simulink model "DDCU_wxt_v02_forA_LabviewV03"  (R2014a)
settings: Solver=FixedStepDiscrete  StartTime=0.0  StopTime=50  FixedStep=0.0005  RelTol=1e-3
InitFcn:
  | Veh_Par_wxt
values from neighbouring files (symbols this model uses):
  ag_thr = 0.4*g    (= 3.924)    [Veh_Par_wxt.m]
  B = 2.25    [Veh_Par_wxt.m]
  bra_pre_em = 12    [Veh_Par_wxt.m]
  bra_pre_gz2 = 12/3    (= 4)    [Veh_Par_wxt.m]
  bra_pre_gz34 = 12/3    (= 4)    [Veh_Par_wxt.m]
  bra_pre_yd = 12/2    (= 6)    [Veh_Par_wxt.m]
  brakepre_dem_data = [0 1 2 3 4 5 6 7 8 9 10 11 12]    [Veh_Par_wxt.m]
  brakeTrq_dem_data = [0 218.198 436.396 654.594 872.792 1090.99 1309.188 1527.386 1745.584 1963.782 2181.98 2400.178 2618.376]    [Veh_Par_wxt.m]
  bratrq_max = 4*2618.376    (= 10473.504)    [Veh_Par_wxt.m]
  eff_tran = 0.75    [Veh_Par_wxt.m]
  G = Mass*g    (= 36297)    [Veh_Par_wxt.m]
  kd1 = 1    [Veh_Par_wxt.m]
  kd2 = 1    [Veh_Par_wxt.m]
  kd3 = 1    [Veh_Par_wxt.m]
  ki1 = 1    [Veh_Par_wxt.m]
  ki2 = 1    [Veh_Par_wxt.m]
  ki3 = 1    [Veh_Par_wxt.m]
  kp1 = 1    [Veh_Par_wxt.m]
  kp2 = 1    [Veh_Par_wxt.m]
  kp3 = 1    [Veh_Par_wxt.m]
  L = 3.12    [Veh_Par_wxt.m]
  premax = 12    [Veh_Par_wxt.m]
  Radius = 0.20    (= 0.2)    [Veh_Par_wxt.m]
  s_opt_yi_add = 0.05    [Veh_Par_wxt.m]
  s_opt_zhuan_add = 0.05    [Veh_Par_wxt.m]
  spd_map_mot = [0 100 200 300 360 400 500 600 700 800 900]*tras_ratio    [Veh_Par_wxt.m]
  spdmax = 900*tras_ratio    (= 5580)    [Veh_Par_wxt.m]
  speed_thr_park = 5/3.6/Radius*30/pi    (= 66.3145596216)    [Veh_Par_wxt.m]
  tras_ratio = 6.2    [Veh_Par_wxt.m]
  trq_map_mot = [1200 1200 1200 1200 1200 1080 864 720 617 540 480]/tras_ratio    [Veh_Par_wxt.m]
  trqmax = 80    [Veh_Par_wxt.m]
  trqmax_yd = 200    [Veh_Par_wxt.m]
  v_thr1_b = 5    [Veh_Par_wxt.m]
  v_thr2_b = 20    [Veh_Par_wxt.m]
  v_thr_park = 5    [Veh_Par_wxt.m]
undefined symbols (not defined in the file or in its folder): DiscIntNeverNeededParam
libraries: simulink x231, ec5744lib x19
(part 9 of 16)

== system DDCU_wxt_v02_forA_LabviewV03/OutputSignalProcess/VCU_MCU2_replace/M4Drive ==
  M4Drive : Inport
  Constant{1..4,6..8} (7 alike) : Constant  Value=0  OutDataTypeStr=uint8
  M4DriveRon : Rounding  Operator=round
  M4Drive_1sat : Saturate  UpperLimit=12  LowerLimit=0
  M4Drive_Convert : DataTypeConversion  OutDataTypeStr=uint8
  M4Drive_Convert1 : DataTypeConversion  OutDataTypeStr=uint32
  M4Drive_D : Product  Inputs=*/
  M4Drive_F : Constant  OutDataTypeStr=single
  M4Drive_L : simulink/Logic and Bit Operations/Bitwise Operator  logicop=AND  UseBitMask=on  BitMask=12  BitMaskRealWorld=Stored Integer
  M4Drive_O : Constant  Value=0  OutDataTypeStr=single
  M4Drive_S : ArithShift  BitShiftNumber=-2
  M4Drive_sat : Saturate  UpperLimit=3  LowerLimit=0
  M4Drive_st : Sum  Inputs=+-
  output1 : Outport
  output2 : Outport  Port=2
  output3 : Outport  Port=3
  output4 : Outport  Port=4
  output5 : Outport  Port=5
  output6 : Outport  Port=6
  output7 : Outport  Port=7
  output8 : Outport  Port=8
  wires:
  M4Drive/1 -> M4Drive_sat/1
  M4Drive_sat/1 -> M4Drive_st/1
  M4Drive_O/1 -> M4Drive_st/2
  M4Drive_st/1 -> M4Drive_D/1
  M4Drive_F/1 -> M4Drive_D/2
  M4Drive_D/1 -> M4DriveRon/1
  M4DriveRon/1 -> M4Drive_S/1
  M4Drive_S/1 -> M4Drive_1sat/1
  M4Drive_1sat/1 -> M4Drive_Convert1/1
  M4Drive_Convert1/1 -> M4Drive_L/1
  M4Drive_L/1 -> M4Drive_Convert/1
  M4Drive_Convert/1 -> output5/1
  Constant1/1 -> output1/1
  Constant2/1 -> output2/1
  Constant3/1 -> output3/1
  Constant4/1 -> output4/1
  Constant6/1 -> output6/1
  Constant7/1 -> output7/1
  Constant8/1 -> output8/1

== system DDCU_wxt_v02_forA_LabviewV03/OutputSignalProcess/VCU_MCU2_replace/M4Enable ==
  M4Enable : Inport
  Constant{1..3,5..8} (7 alike) : Constant  Value=0  OutDataTypeStr=uint8
  M4EnableRon : Rounding  Operator=round
  M4Enable_1sat : Saturate  UpperLimit=192  LowerLimit=0
  M4Enable_Convert : DataTypeConversion  OutDataTypeStr=uint8
  M4Enable_Convert1 : DataTypeConversion  OutDataTypeStr=uint32
  M4Enable_D : Product  Inputs=*/
  M4Enable_F : Constant  OutDataTypeStr=single
  M4Enable_L : simulink/Logic and Bit Operations/Bitwise Operator  logicop=AND  UseBitMask=on  BitMask=192  BitMaskRealWorld=Stored Integer
  M4Enable_O : Constant  Value=0  OutDataTypeStr=single
  M4Enable_S : ArithShift  BitShiftNumber=-6
  M4Enable_sat : Saturate  UpperLimit=3  LowerLimit=0
  M4Enable_st : Sum  Inputs=+-
  output1 : Outport
  output2 : Outport  Port=2
  output3 : Outport  Port=3
  output4 : Outport  Port=4
  output5 : Outport  Port=5
  output6 : Outport  Port=6
  output7 : Outport  Port=7
  output8 : Outport  Port=8
  wires:
  M4Enable/1 -> M4Enable_sat/1
  M4Enable_sat/1 -> M4Enable_st/1
  M4Enable_O/1 -> M4Enable_st/2
  M4Enable_st/1 -> M4Enable_D/1
  M4Enable_F/1 -> M4Enable_D/2
  M4Enable_D/1 -> M4EnableRon/1
  M4EnableRon/1 -> M4Enable_S/1
  M4Enable_S/1 -> M4Enable_1sat/1
  M4Enable_1sat/1 -> M4Enable_Convert1/1
  M4Enable_Convert1/1 -> M4Enable_L/1
  M4Enable_L/1 -> M4Enable_Convert/1
  M4Enable_Convert/1 -> output4/1
  Constant1/1 -> output1/1
  Constant2/1 -> output2/1
  Constant3/1 -> output3/1
  Constant5/1 -> output5/1
  Constant6/1 -> output6/1
  Constant7/1 -> output7/1
  Constant8/1 -> output8/1

== system DDCU_wxt_v02_forA_LabviewV03/OutputSignalProcess/VCU_MCU2_replace/M4Mode ==
  M4Mode : Inport
  Constant{1..4,6..8} (7 alike) : Constant  Value=0  OutDataTypeStr=uint8
  M4ModeRon : Rounding  Operator=round
  M4Mode_1sat : Saturate  UpperLimit=3  LowerLimit=0
  M4Mode_Convert : DataTypeConversion  OutDataTypeStr=uint8
  M4Mode_Convert1 : DataTypeConversion  OutDataTypeStr=uint32
  M4Mode_D : Product  Inputs=*/
  M4Mode_F : Constant  OutDataTypeStr=single
  M4Mode_L : simulink/Logic and Bit Operations/Bitwise Operator  logicop=AND  UseBitMask=on  BitMask=3  BitMaskRealWorld=Stored Integer
  M4Mode_O : Constant  Value=0  OutDataTypeStr=single
  M4Mode_S : ArithShift
  M4Mode_sat : Saturate  UpperLimit=3  LowerLimit=0
  M4Mode_st : Sum  Inputs=+-
  output1 : Outport
  output2 : Outport  Port=2
  output3 : Outport  Port=3
  output4 : Outport  Port=4
  output5 : Outport  Port=5
  output6 : Outport  Port=6
  output7 : Outport  Port=7
  output8 : Outport  Port=8
  wires:
  M4Mode/1 -> M4Mode_sat/1
  M4Mode_sat/1 -> M4Mode_st/1
  M4Mode_O/1 -> M4Mode_st/2
  M4Mode_st/1 -> M4Mode_D/1
  M4Mode_F/1 -> M4Mode_D/2
  M4Mode_D/1 -> M4ModeRon/1
  M4ModeRon/1 -> M4Mode_S/1
  M4Mode_S/1 -> M4Mode_1sat/1
  M4Mode_1sat/1 -> M4Mode_Convert1/1
  M4Mode_Convert1/1 -> M4Mode_L/1
  M4Mode_L/1 -> M4Mode_Convert/1
  M4Mode_Convert/1 -> output5/1
  Constant1/1 -> output1/1
  Constant2/1 -> output2/1
  Constant3/1 -> output3/1
  Constant4/1 -> output4/1
  Constant6/1 -> output6/1
  Constant7/1 -> output7/1
  Constant8/1 -> output8/1

== system DDCU_wxt_v02_forA_LabviewV03/OutputSignalProcess/VCU_MCU2_replace/M4SpeedLimit ==
  M4SpeedLimit : Inport
  Constant{1..6} (6 alike) : Constant  Value=0  OutDataTypeStr=uint8
  M4SpeedLimitBitCov : DataTypeConversion  OutDataTypeStr=uint8
  M4SpeedLimitCOV : DataTypeConversion  OutDataTypeStr=uint8
  M4SpeedLimitRon : Rounding  Operator=round
  M4SpeedLimit_1sat : Saturate  UpperLimit=4095  LowerLimit=0
  M4SpeedLimit_And : simulink/Logic and Bit Operations/Bitwise Operator  logicop=AND  UseBitMask=off  NumInputPorts=2  BitMask=bin2dec('11011001')  BitMaskRealWorld=Stored Integer
  M4SpeedLimit_And_C : Constant  Value=255  OutDataTypeStr=uint32
  M4SpeedLimit_Convert : DataTypeConversion  OutDataTypeStr=uint32
  M4SpeedLimit_D : Product  Inputs=*/
  M4SpeedLimit_D1 : Product  Inputs=*/
  M4SpeedLimit_F : Constant  Value=5  OutDataTypeStr=single
  M4SpeedLimit_L : simulink/Logic and Bit Operations/Bitwise Operator  logicop=AND  UseBitMask=on  BitMask=4095  BitMaskRealWorld=Stored Integer
  M4SpeedLimit_O : Constant  Value=0  OutDataTypeStr=single
  M4SpeedLimit_S : ArithShift
  M4SpeedLimit_sat : Saturate  UpperLimit=20475  LowerLimit=0
  M4SpeedLimit_st : Sum  Inputs=+-
  M4SpeedLimitoutput8_C : Constant  Value=256
  output1 : Outport
  output2 : Outport  Port=2
  output3 : Outport  Port=3
  output4 : Outport  Port=4
  output5 : Outport  Port=5
  output6 : Outport  Port=6
  output7 : Outport  Port=7
  output8 : Outport  Port=8
  wires:
  M4SpeedLimit/1 -> M4SpeedLimit_sat/1
  M4SpeedLimit_sat/1 -> M4SpeedLimit_st/1
  M4SpeedLimit_O/1 -> M4SpeedLimit_st/2
  M4SpeedLimit_st/1 -> M4SpeedLimit_D/1
  M4SpeedLimit_F/1 -> M4SpeedLimit_D/2
  M4SpeedLimit_D/1 -> M4SpeedLimitRon/1
  M4SpeedLimitRon/1 -> M4SpeedLimit_S/1
  M4SpeedLimit_S/1 -> M4SpeedLimit_1sat/1
  M4SpeedLimit_1sat/1 -> M4SpeedLimit_Convert/1
  M4SpeedLimit_Convert/1 -> M4SpeedLimit_L/1
  M4SpeedLimit_L/1 -> M4SpeedLimit_D1/1, M4SpeedLimit_And/1
  M4SpeedLimitoutput8_C/1 -> M4SpeedLimit_D1/2
  M4SpeedLimit_D1/1 -> M4SpeedLimitCOV/1
  M4SpeedLimitCOV/1 -> output8/1
  M4SpeedLimit_And_C/1 -> M4SpeedLimit_And/2
  M4SpeedLimit_And/1 -> M4SpeedLimitBitCov/1
  M4SpeedLimitBitCov/1 -> output7/1
  Constant1/1 -> output1/1
  Constant2/1 -> output2/1
  Constant3/1 -> output3/1
  Constant4/1 -> output4/1
  Constant5/1 -> output5/1
  Constant6/1 -> output6/1

== system DDCU_wxt_v02_forA_LabviewV03/OutputSignalProcess/VCU_MCU2_replace/M4SpeedSet ==
  M4SpeedSet : Inport
  Constant{1..4,7..8} (6 alike) : Constant  Value=0  OutDataTypeStr=uint8
  M4SpeedSetBitCov : DataTypeConversion  OutDataTypeStr=uint8
  M4SpeedSetCOV : DataTypeConversion  OutDataTypeStr=uint8
  M4SpeedSetRon : Rounding  Operator=round
  M4SpeedSet_1sat : Saturate  UpperLimit=65520  LowerLimit=0
  M4SpeedSet_And : simulink/Logic and Bit Operations/Bitwise Operator  logicop=AND  UseBitMask=off  NumInputPorts=2  BitMask=bin2dec('11011001')  BitMaskRealWorld=Stored Integer
  M4SpeedSet_And_C : Constant  Value=255  OutDataTypeStr=uint32
  M4SpeedSet_Convert : DataTypeConversion  OutDataTypeStr=uint32
  M4SpeedSet_D : Product  Inputs=*/
  M4SpeedSet_D1 : Product  Inputs=*/
  M4SpeedSet_F : Constant  Value=5  OutDataTypeStr=single
  M4SpeedSet_L : simulink/Logic and Bit Operations/Bitwise Operator  logicop=AND  UseBitMask=on  BitMask=65520  BitMaskRealWorld=Stored Integer
  M4SpeedSet_O : Constant  Value=-5000  OutDataTypeStr=single
  M4SpeedSet_S : ArithShift  BitShiftNumber=-4
  M4SpeedSet_sat : Saturate  UpperLimit=15475  LowerLimit=-5000
  M4SpeedSet_st : Sum  Inputs=+-
  M4SpeedSetoutput6_C : Constant  Value=256
  output1 : Outport
  output2 : Outport  Port=2
  output3 : Outport  Port=3
  output4 : Outport  Port=4
  output5 : Outport  Port=5
  output6 : Outport  Port=6
  output7 : Outport  Port=7
  output8 : Outport  Port=8
  wires:
  M4SpeedSet/1 -> M4SpeedSet_sat/1
  M4SpeedSet_sat/1 -> M4SpeedSet_st/1
  M4SpeedSet_O/1 -> M4SpeedSet_st/2
  M4SpeedSet_st/1 -> M4SpeedSet_D/1
  M4SpeedSet_F/1 -> M4SpeedSet_D/2
  M4SpeedSet_D/1 -> M4SpeedSetRon/1
  M4SpeedSetRon/1 -> M4SpeedSet_S/1
  M4SpeedSet_S/1 -> M4SpeedSet_1sat/1
  M4SpeedSet_1sat/1 -> M4SpeedSet_Convert/1
  M4SpeedSet_Convert/1 -> M4SpeedSet_L/1
  M4SpeedSet_L/1 -> M4SpeedSet_D1/1, M4SpeedSet_And/1
  M4SpeedSetoutput6_C/1 -> M4SpeedSet_D1/2
  M4SpeedSet_D1/1 -> M4SpeedSetCOV/1
  M4SpeedSetCOV/1 -> output6/1
  M4SpeedSet_And_C/1 -> M4SpeedSet_And/2
  M4SpeedSet_And/1 -> M4SpeedSetBitCov/1
  M4SpeedSetBitCov/1 -> output5/1
  Constant1/1 -> output1/1
  Constant2/1 -> output2/1
  Constant3/1 -> output3/1
  Constant4/1 -> output4/1
  Constant7/1 -> output7/1
  Constant8/1 -> output8/1

== system DDCU_wxt_v02_forA_LabviewV03/OutputSignalProcess/VCU_MCU2_replace/MCU2HeartBeat ==
  MCU2HeartBeat : Inport
  Constant{1..7} (7 alike) : Constant  Value=0  OutDataTypeStr=uint8
  MCU2HeartBeatRon : Rounding  Operator=round
  MCU2HeartBeat_1sat : Saturate  UpperLimit=240  LowerLimit=0
  MCU2HeartBeat_Convert : DataTypeConversion  OutDataTypeStr=uint8
  MCU2HeartBeat_Convert1 : DataTypeConversion  OutDataTypeStr=uint32
  MCU2HeartBeat_D : Product  Inputs=*/
  MCU2HeartBeat_F : Constant  OutDataTypeStr=single
  MCU2HeartBeat_L : simulink/Logic and Bit Operations/Bitwise Operator  logicop=AND  UseBitMask=on  BitMask=240  BitMaskRealWorld=Stored Integer
  MCU2HeartBeat_O : Constant  Value=0  OutDataTypeStr=single
  MCU2HeartBeat_S : ArithShift  BitShiftNumber=-4
  MCU2HeartBeat_sat : Saturate  UpperLimit=15  LowerLimit=0
  MCU2HeartBeat_st : Sum  Inputs=+-
  output1 : Outport
  output2 : Outport  Port=2
  output3 : Outport  Port=3
  output4 : Outport  Port=4
  output5 : Outport  Port=5
  output6 : Outport  Port=6
  output7 : Outport  Port=7
  output8 : Outport  Port=8
  wires:
  MCU2HeartBeat/1 -> MCU2HeartBeat_sat/1
  MCU2HeartBeat_sat/1 -> MCU2HeartBeat_st/1
  MCU2HeartBeat_O/1 -> MCU2HeartBeat_st/2
  MCU2HeartBeat_st/1 -> MCU2HeartBeat_D/1
  MCU2HeartBeat_F/1 -> MCU2HeartBeat_D/2
  MCU2HeartBeat_D/1 -> MCU2HeartBeatRon/1
  MCU2HeartBeatRon/1 -> MCU2HeartBeat_S/1
  MCU2HeartBeat_S/1 -> MCU2HeartBeat_1sat/1
  MCU2HeartBeat_1sat/1 -> MCU2HeartBeat_Convert1/1
  MCU2HeartBeat_Convert1/1 -> MCU2HeartBeat_L/1
  MCU2HeartBeat_L/1 -> MCU2HeartBeat_Convert/1
  MCU2HeartBeat_Convert/1 -> output8/1
  Constant1/1 -> output1/1
  Constant2/1 -> output2/1
  Constant3/1 -> output3/1
  Constant4/1 -> output4/1
  Constant5/1 -> output5/1
  Constant6/1 -> output6/1
  Constant7/1 -> output7/1

== system DDCU_wxt_v02_forA_LabviewV03/OutputSignalProcess/VCU_Park/ParkEnable ==
  ParkEnable : Inport
  Constant{2..8} (7 alike) : Constant  Value=0  OutDataTypeStr=uint8
  ParkEnableRon : Rounding  Operator=round
  ParkEnable_1sat : Saturate  UpperLimit=1  LowerLimit=0
  ParkEnable_Convert : DataTypeConversion  OutDataTypeStr=uint8
  ParkEnable_Convert1 : DataTypeConversion  OutDataTypeStr=uint32
  ParkEnable_D : Product  Inputs=*/
  ParkEnable_F : Constant  OutDataTypeStr=single
  ParkEnable_L : simulink/Logic and Bit Operations/Bitwise Operator  logicop=AND  UseBitMask=on  BitMask=1  BitMaskRealWorld=Stored Integer
  ParkEnable_O : Constant  Value=0  OutDataTypeStr=single
  ParkEnable_S : ArithShift
  ParkEnable_sat : Saturate  UpperLimit=1  LowerLimit=0
  ParkEnable_st : Sum  Inputs=+-
  output1 : Outport
  output2 : Outport  Port=2
  output3 : Outport  Port=3
  output4 : Outport  Port=4
  output5 : Outport  Port=5
  output6 : Outport  Port=6
  output7 : Outport  Port=7
  output8 : Outport  Port=8
  wires:
  ParkEnable/1 -> ParkEnable_sat/1
  ParkEnable_sat/1 -> ParkEnable_st/1
  ParkEnable_O/1 -> ParkEnable_st/2
  ParkEnable_st/1 -> ParkEnable_D/1
  ParkEnable_F/1 -> ParkEnable_D/2
  ParkEnable_D/1 -> ParkEnableRon/1
  ParkEnableRon/1 -> ParkEnable_S/1
  ParkEnable_S/1 -> ParkEnable_1sat/1
  ParkEnable_1sat/1 -> ParkEnable_Convert1/1
  ParkEnable_Convert1/1 -> ParkEnable_L/1
  ParkEnable_L/1 -> ParkEnable_Convert/1
  ParkEnable_Convert/1 -> output1/1
  Constant2/1 -> output2/1
  Constant3/1 -> output3/1
  Constant4/1 -> output4/1
  Constant5/1 -> output5/1
  Constant6/1 -> output6/1
  Constant7/1 -> output7/1
  Constant8/1 -> output8/1

== system DDCU_wxt_v02_forA_LabviewV03/Data_Input/Function-Call Subsystem/ddcu1_ddcu2/acc_dem_Sub ==
  In1 : Inport
  Out1 : Outport
  wires:
  In1/1 -> Out1/1

== system DDCU_wxt_v02_forA_LabviewV03/Data_Input/Function-Call Subsystem/ddcu1_ddcu2/brake_dem_Sub ==
  In1 : Inport
  Out1 : Outport
  wires:
  In1/1 -> Out1/1

== system DDCU_wxt_v02_forA_LabviewV03/Data_Input/Function-Call Subsystem/ddcu1_ddcu2/brake_emerg_Sub ==
  In1 : Inport
  Out1 : Outport
  wires:
  In1/1 -> Out1/1

== system DDCU_wxt_v02_forA_LabviewV03/Data_Input/Function-Call Subsystem/ddcu1_ddcu2/mode_dem_Sub ==
  In1 : Inport
  Out1 : Outport
  wires:
  In1/1 -> Out1/1

== system DDCU_wxt_v02_forA_LabviewV03/Data_Input/Function-Call Subsystem/ddcu1_ddcu2/steer_dem_Sub ==
  In1 : Inport
  Out1 : Outport
  wires:
  In1/1 -> Out1/1

== system DDCU_wxt_v02_forA_LabviewV03/Data_Input/Function-Call Subsystem2/ESC_VCU/VESC_BrkFlt_enum_Sub ==
  In1 : Inport
  Out1 : Outport
  wires:
  In1/1 -> Out1/1

== system DDCU_wxt_v02_forA_LabviewV03/Data_Input/Function-Call Subsystem2/ESC_VCU/VESC_BrkPLe_MPa_Sub ==
  In1 : Inport
  Out1 : Outport
  wires:
  In1/1 -> Out1/1

== system DDCU_wxt_v02_forA_LabviewV03/Data_Input/Function-Call Subsystem2/ESC_VCU/VESC_BrkPMa_MPa_Sub ==
  In1 : Inport
  Out1 : Outport
  wires:
  In1/1 -> Out1/1

== system DDCU_wxt_v02_forA_LabviewV03/Data_Input/Function-Call Subsystem2/ESC_VCU/VESC_BrkPRi_MPa_Sub ==
  In1 : Inport
  Out1 : Outport
  wires:
  In1/1 -> Out1/1

== system DDCU_wxt_v02_forA_LabviewV03/Data_Input/Function-Call Subsystem2/ESC_VCU/VESC_BrkPSetLe_MPa_Sub ==
  In1 : Inport
  Out1 : Outport
  wires:
  In1/1 -> Out1/1

== system DDCU_wxt_v02_forA_LabviewV03/Data_Input/Function-Call Subsystem2/ESC_VCU/VESC_BrkPSetRi_MPa_Sub ==
  In1 : Inport
  Out1 : Outport
  wires:
  In1/1 -> Out1/1

== system DDCU_wxt_v02_forA_LabviewV03/Data_Input/Function-Call Subsystem2/ESC_VCU/VESC_BrkReq_flg_Sub ==
  In1 : Inport
  Out1 : Outport
  wires:
  In1/1 -> Out1/1

== system DDCU_wxt_v02_forA_LabviewV03/Data_Input/Function-Call Subsystem2/ESC_VCU/VESC_HotSts_flg_Sub ==
  In1 : Inport
  Out1 : Outport
  wires:
  In1/1 -> Out1/1

== system DDCU_wxt_v02_forA_LabviewV03/Data_Input/Function-Call Subsystem2/ESC_VCU/VESC_ParkReq_flg_Sub ==
  In1 : Inport
  Out1 : Outport
  wires:
  In1/1 -> Out1/1

== system DDCU_wxt_v02_forA_LabviewV03/Data_Input/HCU1_VCU/HCU1_VCU/acc_Sub ==
  In1 : Inport
  Out1 : Outport
  wires:
  In1/1 -> Out1/1

== system DDCU_wxt_v02_forA_LabviewV03/Data_Input/HCU1_VCU/HCU1_VCU/break_Sub ==
  In1 : Inport
  Out1 : Outport
  wires:
  In1/1 -> Out1/1

== system DDCU_wxt_v02_forA_LabviewV03/Data_Input/HCU1_VCU/HCU1_VCU/pwr_limit_Sub ==
  In1 : Inport
  Out1 : Outport
  wires:
  In1/1 -> Out1/1

== system DDCU_wxt_v02_forA_LabviewV03/Data_Input/HCU1_VCU/HCU1_VCU/real_velocity_Sub ==
  In1 : Inport
  Out1 : Outport
  wires:
  In1/1 -> Out1/1

== system DDCU_wxt_v02_forA_LabviewV03/Data_Input/HCU1_VCU/HCU1_VCU/turn_Sub ==
  In1 : Inport
  Out1 : Outport
  wires:
  In1/1 -> Out1/1

== system DDCU_wxt_v02_forA_LabviewV03/Data_Input/HCU1_VCU1/MUC1_VCU1/spd_mot_lf_Sub ==
  In1 : Inport
  Out1 : Outport
  wires:
  In1/1 -> Out1/1

== system DDCU_wxt_v02_forA_LabviewV03/Data_Input/HCU1_VCU1/MUC1_VCU1/spd_mot_lr_Sub ==
  In1 : Inport
  Out1 : Outport
  wires:
  In1/1 -> Out1/1

== system DDCU_wxt_v02_forA_LabviewV03/Data_Input/HCU1_VCU1/MUC1_VCU1/spd_mot_rf_Sub ==
  In1 : Inport
  Out1 : Outport
  wires:
  In1/1 -> Out1/1

== system DDCU_wxt_v02_forA_LabviewV03/Data_Input/HCU1_VCU1/MUC1_VCU1/spd_mot_rr_Sub ==
  In1 : Inport
  Out1 : Outport
  wires:
  In1/1 -> Out1/1

== system DDCU_wxt_v02_forA_LabviewV03/Data_Input/HCU2_VCU/HCU2_VCU/daodang_Sub ==
  In1 : Inport
  Out1 : Outport
  wires:
  In1/1 -> Out1/1

== system DDCU_wxt_v02_forA_LabviewV03/Data_Input/HCU2_VCU/HCU2_VCU/kongdang_Sub ==
  In1 : Inport
  Out1 : Outport
  wires:
  In1/1 -> Out1/1

== system DDCU_wxt_v02_forA_LabviewV03/Data_Input/HCU2_VCU/HCU2_VCU/qianjin_Sub ==
  In1 : Inport
  Out1 : Outport
  wires:
  In1/1 -> Out1/1

== system DDCU_wxt_v02_forA_LabviewV03/Data_Input/HCU2_VCU/HCU2_VCU/zhongxinzhuanxiang_Sub ==
  In1 : Inport
  Out1 : Outport
  wires:
  In1/1 -> Out1/1

== system DDCU_wxt_v02_forA_LabviewV03/Data_Input/HCU2_VCU/HCU2_VCU/zhuche_Sub ==
  In1 : Inport
  Out1 : Outport
  wires:
  In1/1 -> Out1/1

== system DDCU_wxt_v02_forA_LabviewV03/Data_Input/MCU1_VCU1/MCU1_VCU1/M1Current_Sub ==
  In1 : Inport
  Out1 : Outport
  wires:
  In1/1 -> Out1/1

== system DDCU_wxt_v02_forA_LabviewV03/Data_Input/MCU1_VCU1/MCU1_VCU1/M1Direction_Sub ==
  In1 : Inport
  Out1 : Outport
  wires:
  In1/1 -> Out1/1

== system DDCU_wxt_v02_forA_LabviewV03/Data_Input/MCU1_VCU1/MCU1_VCU1/M1HeartBeat_Sub ==
  In1 : Inport
  Out1 : Outport
  wires:
  In1/1 -> Out1/1

== system DDCU_wxt_v02_forA_LabviewV03/Data_Input/MCU1_VCU1/MCU1_VCU1/M1InputVolt_Sub ==
  In1 : Inport
  Out1 : Outport
  wires:
  In1/1 -> Out1/1

== system DDCU_wxt_v02_forA_LabviewV03/Data_Input/MCU1_VCU1/MCU1_VCU1/M1Speed_Sub ==
  In1 : Inport
  Out1 : Outport
  wires:
  In1/1 -> Out1/1

== system DDCU_wxt_v02_forA_LabviewV03/Data_Input/MCU1_VCU1/MCU1_VCU1/M1State_Sub ==
  In1 : Inport
  Out1 : Outport
  wires:
  In1/1 -> Out1/1

== system DDCU_wxt_v02_forA_LabviewV03/Data_Input/MCU1_VCU1/MCU1_VCU1/M1Torque_Sub ==
  In1 : Inport
  Out1 : Outport
  wires:
  In1/1 -> Out1/1

== system DDCU_wxt_v02_forA_LabviewV03/Data_Input/MCU1_VCU2/MCU1_VCU2/M1FaultCode_Sub ==
  In1 : Inport
  Out1 : Outport
  wires:
  In1/1 -> Out1/1

== system DDCU_wxt_v02_forA_LabviewV03/Data_Input/MCU1_VCU2/MCU1_VCU2/M1FaultGrade_Sub ==
  In1 : Inport
  Out1 : Outport
  wires:
  In1/1 -> Out1/1

== system DDCU_wxt_v02_forA_LabviewV03/Data_Input/MCU1_VCU2/MCU1_VCU2/M1IGBTTemp_Sub ==
  In1 : Inport
  Out1 : Outport
  wires:
  In1/1 -> Out1/1

== system DDCU_wxt_v02_forA_LabviewV03/Data_Input/MCU1_VCU2/MCU1_VCU2/M1Temp_Sub ==
  In1 : Inport
  Out1 : Outport
  wires:
  In1/1 -> Out1/1

== system DDCU_wxt_v02_forA_LabviewV03/Data_Input/MCU1_VCU2/MCU1_VCU2/M1TqLimit_Sub ==
  In1 : Inport
  Out1 : Outport
  wires:
  In1/1 -> Out1/1

== system DDCU_wxt_v02_forA_LabviewV03/Data_Input/MCU1_VCU3/MCU1_VCU3/M2Current_Sub ==
  In1 : Inport
  Out1 : Outport
  wires:
  In1/1 -> Out1/1

== system DDCU_wxt_v02_forA_LabviewV03/Data_Input/MCU1_VCU3/MCU1_VCU3/M2Direction_Sub ==
  In1 : Inport
  Out1 : Outport
  wires:
  In1/1 -> Out1/1

== system DDCU_wxt_v02_forA_LabviewV03/Data_Input/MCU1_VCU3/MCU1_VCU3/M2HeartBeat_Sub ==
  In1 : Inport
  Out1 : Outport
  wires:
  In1/1 -> Out1/1

== system DDCU_wxt_v02_forA_LabviewV03/Data_Input/MCU1_VCU3/MCU1_VCU3/M2InputVolt_Sub ==
  In1 : Inport
  Out1 : Outport
  wires:
  In1/1 -> Out1/1

== system DDCU_wxt_v02_forA_LabviewV03/Data_Input/MCU1_VCU3/MCU1_VCU3/M2Speed_Sub ==
  In1 : Inport
  Out1 : Outport
  wires:
  In1/1 -> Out1/1

== system DDCU_wxt_v02_forA_LabviewV03/Data_Input/MCU1_VCU3/MCU1_VCU3/M2State_Sub ==
  In1 : Inport
  Out1 : Outport
  wires:
  In1/1 -> Out1/1

== system DDCU_wxt_v02_forA_LabviewV03/Data_Input/MCU1_VCU3/MCU1_VCU3/M2Torque_Sub ==
  In1 : Inport
  Out1 : Outport
  wires:
  In1/1 -> Out1/1

== system DDCU_wxt_v02_forA_LabviewV03/Data_Input/MCU1_VCU4/MCU1_VCU4/M2FaultCode_Sub ==
  In1 : Inport
  Out1 : Outport
  wires:
  In1/1 -> Out1/1

== system DDCU_wxt_v02_forA_LabviewV03/Data_Input/MCU1_VCU4/MCU1_VCU4/M2FaultGrade_Sub ==
  In1 : Inport
  Out1 : Outport
  wires:
  In1/1 -> Out1/1

== system DDCU_wxt_v02_forA_LabviewV03/Data_Input/MCU1_VCU4/MCU1_VCU4/M2IGBTTemp_Sub ==
  In1 : Inport
  Out1 : Outport
  wires:
  In1/1 -> Out1/1

== system DDCU_wxt_v02_forA_LabviewV03/Data_Input/MCU1_VCU4/MCU1_VCU4/M2Temp_Sub ==
  In1 : Inport
  Out1 : Outport
  wires:
  In1/1 -> Out1/1

== system DDCU_wxt_v02_forA_LabviewV03/Data_Input/MCU1_VCU4/MCU1_VCU4/M2TqLimit_Sub ==
  In1 : Inport
  Out1 : Outport
  wires:
  In1/1 -> Out1/1

== system DDCU_wxt_v02_forA_LabviewV03/Data_Input/MCU2_VCU1/MCU2_VCU1/M3Current_Sub ==
  In1 : Inport
  Out1 : Outport
  wires:
  In1/1 -> Out1/1

== system DDCU_wxt_v02_forA_LabviewV03/Data_Input/MCU2_VCU1/MCU2_VCU1/M3Direction_Sub ==
  In1 : Inport
  Out1 : Outport
  wires:
  In1/1 -> Out1/1

== system DDCU_wxt_v02_forA_LabviewV03/Data_Input/MCU2_VCU1/MCU2_VCU1/M3HeartBeat_Sub ==
  In1 : Inport
  Out1 : Outport
  wires:
  In1/1 -> Out1/1

== matlab function DDCU_wxt_v02_forA_LabviewV03/MainControl/mode_control/emergency_stop/emergency_stop/HeartBeat1 ==
  data: life_pre input; life output
function life = fcn(life_pre)
%#codegen
life=life_pre+1;
if life>15
    life=0;
end
end

== matlab function DDCU_wxt_v02_forA_LabviewV03/MainControl/mode_control/backward/backward/Brake/MATLAB Function3 ==
  data: syi_act_rf input; flagyi_rf output; s_opt_yi input; s_opt_yi_add input; flagyi_rf_pre input
function flagyi_rf = fcn(syi_act_rf,s_opt_yi,s_opt_yi_add,flagyi_rf_pre)
%#codegen
if syi_act_rf>s_opt_yi+s_opt_yi_add
    flagyi_rf=1;
elseif syi_act_rf<s_opt_yi
    flagyi_rf = 0;
else
    flagyi_rf=flagyi_rf_pre;
end
end

== matlab function DDCU_wxt_v02_forA_LabviewV03/MainControl/mode_control/backward/backward/Drive/驱动防滑控制TCS/MATLAB Function ==
  data: steer_dem input; y output
function y = fcn(steer_dem)
%#codegen 如果有转向，y=0,无转向，y=1
if steer_dem~=0
y = 0;
else y=1;
end
end

== matlab function DDCU_wxt_v02_forA_LabviewV03/MainControl/mode_control/backward/backward/Drive/驱动防滑控制TCS/直行TCS/直行/MATLAB Function ==
  data: s_act_lf input; flag_lf output; s_opt_zhuan input; s_opt_zhuan_add input; flag_lf_pre input
function flag_lf = fcn(s_act_lf,s_opt_zhuan,s_opt_zhuan_add,flag_lf_pre)
%#codegen
if s_act_lf>s_opt_zhuan+s_opt_zhuan_add
    flag_lf=1;
elseif s_act_lf<s_opt_zhuan
    flag_lf = 0;
else
    flag_lf=flag_lf_pre;
end
end

== matlab function DDCU_wxt_v02_forA_LabviewV03/MainControl/mode_control/backward/backward/Drive/驱动防滑控制TCS/转向TCS/右转/MATLAB Function1 ==
  data: s_act_lr input; flag_lr output; s_opt_zhuan input; s_opt_zhuan_add input; flag_lr_pre input
function flag_lr = fcn(s_act_lr,s_opt_zhuan,s_opt_zhuan_add,flag_lr_pre)
%#codegen
if s_act_lr>s_opt_zhuan+s_opt_zhuan_add
    flag_lr=1;
elseif s_act_lr<s_opt_zhuan
    flag_lr = 0;
else
    flag_lr=flag_lr_pre;
end
end

== matlab function DDCU_wxt_v02_forA_LabviewV03/MainControl/mode_control/backward/backward/Drive/驱动防滑控制TCS/转向TCS/右转/前轮滑转/HeartBeat1 ==
  data: life_pre input; life output
function life = fcn(life_pre)
%#codegen
life=life_pre+1;
if life>15
    life=0;
end
end

== matlab function DDCU_wxt_v02_forA_LabviewV03/MainControl/mode_control/backward/backward/Drive/驱动防滑控制TCS/转向TCS/左转/MATLAB Function1 ==
  data: s_act_lr input; flag_lr output; s_opt_zhuan input; s_opt_zhuan_add input; flag_lr_pre input
function flag_lr = fcn(s_act_lr,s_opt_zhuan,s_opt_zhuan_add,flag_lr_pre)
%#codegen
if s_act_lr>s_opt_zhuan+s_opt_zhuan_add
    flag_lr=1;
elseif s_act_lr<s_opt_zhuan
    flag_lr = 0;
else
    flag_lr=flag_lr_pre;
end
end

== matlab function DDCU_wxt_v02_forA_LabviewV03/MainControl/mode_control/backward/backward/Drive/驱动防滑控制TCS/转向TCS/左转/前轮滑转/HeartBeat ==
  data: life_pre input; life output
function life = fcn(life_pre)
%#codegen
life=life_pre+1;
if life>15
    life=0;
end
end
